simulink model "simulink_controller_3"  (R2020a)
settings: Solver=VariableStepAuto  StartTime=0.0  StopTime=10.0  RelTol=1e-3
libraries: simulink x2
settings Model: Creator=Jordan  LastModifiedBy=Jordan

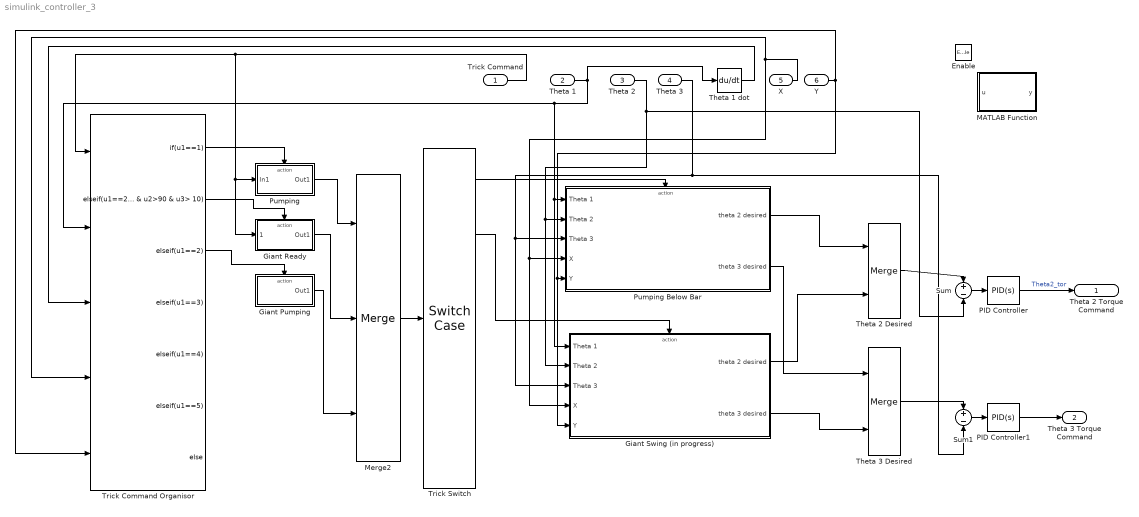
== system simulink_controller_3 ==
  "Trick Command " : Inport
  Theta 1 : Inport  Port=2
  Theta 2 : Inport  Port=3
  Theta 3 : Inport  Port=4
  X : Inport  Port=5
  Y : Inport  Port=6
  Enable : EnablePort
  Giant Pumping : Subsystem  TreatAsAtomicUnit=on
  Giant Ready : Subsystem  TreatAsAtomicUnit=on
  Giant Swing (in progress) : Subsystem  TreatAsAtomicUnit=on
  MATLAB Function : MATLAB Function  TreatAsAtomicUnit=on
  Merge2 : Merge  Inputs=3
  PID Controller : simulink/Continuous/PID Controller  Controller=PID  Form=Parallel  TimeDomain=Continuous-time  UseExternalTs=off  SampleTime=-1  IntegratorMethod=Forward Euler  FilterMethod=Forward Euler  ControllerParametersSource=internal  P=1  I=1  D=0  UseFilter=on  N=100  TunerSelectOption=Transfer Function Based (PID Tuner App)  InitialConditionSource=internal  InitialConditionForIntegrator=0  InitialConditionForFilter=0  DifferentiatorICPrevScaledInput=0  ExternalReset=none  TrackingMode=off  Kt=1  LimitOutput=off  UpperSaturationLimit=inf  LowerSaturationLimit=-inf  LinearizeAsGain=on  AntiWindupMode=none  Kb=1  POutMin=[]  POutMax=[]  IOutMin=[]  IOutMax=[]  DOutMin=[]  DOutMax=[]  NOutMin=[]  NOutMax=[]  SumOutMin=[]  SumOutMax=[]  SaturationOutMin=[]  SaturationOutMax=[]  PParamMin=[]  PParamMax=[]  IParamMin=[]  IParamMax=[]  DParamMin=[]  DParamMax=[]  NParamMin=[]  NParamMax=[]  KbParamMin=[]  KbParamMax=[]  KtParamMin=[]  KtParamMax=[]  KbOutMin=[]  KbOutMax=[]  KtOutMin=[]  KtOutMax=[]  IntegratorOutMin=[]  IntegratorOutMax=[]  FilterOutMin=[]  FilterOutMax=[]  SumI1OutMin=[]  SumI1OutMax=[]  SumI2OutMin=[]  SumI2OutMax=[]  SumI3OutMin=[]  SumI3OutMax=[]  SumI4OutMin=[]  SumI4OutMax=[]  SumDOutMin=[]  SumDOutMax=[]  DifferentiatorOutMin=[]  DifferentiatorOutMax=[]  FilterDiffOutCoefMin=[]  FilterDiffOutCoefMax=[]  ReciprocalOutMin=[]  ReciprocalOutMax=[]  SumDenOutMin=[]  SumDenOutMax=[]  SumNumOutMin=[]  SumNumOutMax=[]  DivideOutMin=[]  DivideOutMax=[]  UdiffTsProdOutMin=[]  UdiffTsProdOutMax=[]  NTsProdOutMin=[]  NTsProdOutMax=[]  UintegralTsProdOutMin=[]  UintegralTsProdOutMax=[]  UngainTsProdOutMin=[]  UngainTsProdOutMax=[]  IntegratorContinuousStateAttributes=''  IntegratorStateMustResolveToSignalObject=off  IntegratorRTWStateStorageClass=Auto  FilterContinuousStateAttributes=''  FilterStateMustResolveToSignalObject=off  FilterRTWStateStorageClass=Auto  ParallelPVariant=InternalParameters  IdealPVariant=Disabled  IVariant=InternalParameters  DVariant=InternalParameters  IntegratorVariant=Continuous  SatVariant=Disabled  AWVariant=Passthrough  PCopyVariant=Disabled  TRVariant=Disabled  FdbkBlocksVariant=Forward  IdealPFdbkVariant=Disabled  SatFdbkVariant=Disabled  DerivativeFilterVariant=ContFilter  NVariant=InternalParameters  NCopyVariant=Disabled  FilterICVariant=InternalICsFilter  IntegratorICVariant=InternalICs  ExternalResetVariant=Disabled  TRSumVariant=Passthrough  SumFdbkVariant=Disabled  SumVariant=Sum_PID  TsampFilterVariant=InternalTs  TsampNgainVariant=Passthrough  TsampIntegralVariant=Passthrough
  PID Controller1 : simulink/Continuous/PID Controller  Controller=PID  Form=Parallel  TimeDomain=Continuous-time  UseExternalTs=off  SampleTime=-1  IntegratorMethod=Forward Euler  FilterMethod=Forward Euler  ControllerParametersSource=internal  P=1  I=1  D=0  UseFilter=on  N=100  TunerSelectOption=Transfer Function Based (PID Tuner App)  InitialConditionSource=internal  InitialConditionForIntegrator=0  InitialConditionForFilter=0  DifferentiatorICPrevScaledInput=0  ExternalReset=none  TrackingMode=off  Kt=1  LimitOutput=off  UpperSaturationLimit=inf  LowerSaturationLimit=-inf  LinearizeAsGain=on  AntiWindupMode=none  Kb=1  POutMin=[]  POutMax=[]  IOutMin=[]  IOutMax=[]  DOutMin=[]  DOutMax=[]  NOutMin=[]  NOutMax=[]  SumOutMin=[]  SumOutMax=[]  SaturationOutMin=[]  SaturationOutMax=[]  PParamMin=[]  PParamMax=[]  IParamMin=[]  IParamMax=[]  DParamMin=[]  DParamMax=[]  NParamMin=[]  NParamMax=[]  KbParamMin=[]  KbParamMax=[]  KtParamMin=[]  KtParamMax=[]  KbOutMin=[]  KbOutMax=[]  KtOutMin=[]  KtOutMax=[]  IntegratorOutMin=[]  IntegratorOutMax=[]  FilterOutMin=[]  FilterOutMax=[]  SumI1OutMin=[]  SumI1OutMax=[]  SumI2OutMin=[]  SumI2OutMax=[]  SumI3OutMin=[]  SumI3OutMax=[]  SumI4OutMin=[]  SumI4OutMax=[]  SumDOutMin=[]  SumDOutMax=[]  DifferentiatorOutMin=[]  DifferentiatorOutMax=[]  FilterDiffOutCoefMin=[]  FilterDiffOutCoefMax=[]  ReciprocalOutMin=[]  ReciprocalOutMax=[]  SumDenOutMin=[]  SumDenOutMax=[]  SumNumOutMin=[]  SumNumOutMax=[]  DivideOutMin=[]  DivideOutMax=[]  UdiffTsProdOutMin=[]  UdiffTsProdOutMax=[]  NTsProdOutMin=[]  NTsProdOutMax=[]  UintegralTsProdOutMin=[]  UintegralTsProdOutMax=[]  UngainTsProdOutMin=[]  UngainTsProdOutMax=[]  IntegratorContinuousStateAttributes=''  IntegratorStateMustResolveToSignalObject=off  IntegratorRTWStateStorageClass=Auto  FilterContinuousStateAttributes=''  FilterStateMustResolveToSignalObject=off  FilterRTWStateStorageClass=Auto  ParallelPVariant=InternalParameters  IdealPVariant=Disabled  IVariant=InternalParameters  DVariant=InternalParameters  IntegratorVariant=Continuous  SatVariant=Disabled  AWVariant=Passthrough  PCopyVariant=Disabled  TRVariant=Disabled  FdbkBlocksVariant=Forward  IdealPFdbkVariant=Disabled  SatFdbkVariant=Disabled  DerivativeFilterVariant=ContFilter  NVariant=InternalParameters  NCopyVariant=Disabled  FilterICVariant=InternalICsFilter  IntegratorICVariant=InternalICs  ExternalResetVariant=Disabled  TRSumVariant=Passthrough  SumFdbkVariant=Disabled  SumVariant=Sum_PID  TsampFilterVariant=InternalTs  TsampNgainVariant=Passthrough  TsampIntegralVariant=Passthrough
  Pumping : Subsystem  TreatAsAtomicUnit=on
  Pumping Below Bar : Subsystem  TreatAsAtomicUnit=on
  Sum : Sum  Inputs=+-
  Sum1 : Sum  Inputs=+-
  Theta 1 dot : Derivative
  Theta 2 Desired : Merge
  Theta 3 Desired : Merge
  Trick Command Organisor : If  NumInputs=5  IfExpression=u1==1  ElseIfExpressions=u1==2 & u2>90 & u3> 10, u1==2, u1==3, u1==4, u1==5
  Trick Switch : SwitchCase  CaseConditions={1,2,3,4,5}
  Theta 2 Torque Command : Outport
  Theta 3 Torque Command : Outport  Port=2
  wires:
  Theta 2 Desired/1 -> Sum/1
  Theta 3 Desired/1 -> Sum1/1
  Giant Swing (in progress)/1(theta 2 desired) -> Theta 2 Desired/2
  Trick Switch/2 -> Giant Swing (in progress)/Action
  Pumping Below Bar/2(theta 3 desired) -> Theta 3 Desired/1
  Giant Swing (in progress)/2(theta 3 desired) -> Theta 3 Desired/2
  Pumping Below Bar/1(theta 2 desired) -> Theta 2 Desired/1
  Trick Switch/1 -> Pumping Below Bar/Action
  "Trick Command "/1 -> Giant Ready/1(" "), Pumping/1(In1), Trick Command Organisor/1
  Theta 2/1 -> Sum/2, Giant Swing (in progress)/2(Theta 2), Pumping Below Bar/2(Theta 2)
  Theta 3/1 -> Sum1/2, Pumping Below Bar/3(Theta 3), Giant Swing (in progress)/3(Theta 3)
  X/1 -> Trick Command Organisor/4, Giant Swing (in progress)/4(X), Pumping Below Bar/4(X)
  Y/1 -> Trick Command Organisor/5, Giant Swing (in progress)/5(Y), Pumping Below Bar/5(Y)
  Theta 1/1 -> Giant Swing (in progress)/1(Theta 1), Pumping Below Bar/1(Theta 1), Trick Command Organisor/2, Theta 1 dot/1
  Theta 1 dot/1 -> Trick Command Organisor/3
  Merge2/1 -> Trick Switch/1
  Trick Command Organisor/1 -> Pumping/Action
  Pumping/1(Out1) -> Merge2/1
  Trick Command Organisor/2 -> Giant Ready/Action
  Giant Ready/1(Out1) -> Merge2/2
  Trick Command Organisor/3 -> Giant Pumping/Action
  Giant Pumping/1(Out1) -> Merge2/3
  PID Controller/1 -> Theta 2 Torque Command/1  "Theta2_tor"
  PID Controller1/1 -> Theta 3 Torque Command/1
  Sum/1 -> PID Controller/1
  Sum1/1 -> PID Controller1/1
  ? -> ?

== system simulink_controller_3/Giant Pumping ==
  Action Port : ActionPort  ActionPortLabel=elseif( u1==2)
  Constant : Constant
  Out1 : Outport
  wires:
  Constant/1 -> Out1/1

== system simulink_controller_3/Giant Ready ==
  " " : Inport
  Action Port : ActionPort  ActionPortLabel=elseif(u1==2 & u2>90 & u3> 10)
  Out1 : Outport
  wires:
  " "/1 -> Out1/1

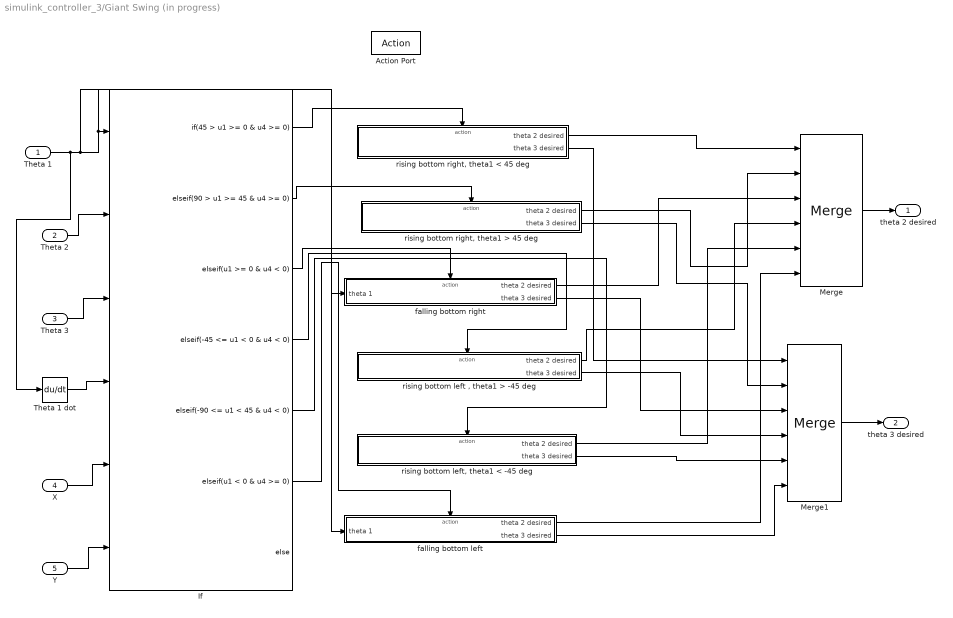
== system simulink_controller_3/Giant Swing (in progress) ==
  Theta 1 : Inport
  Theta 2 : Inport  Port=2
  Theta 3 : Inport  Port=3
  X : Inport  Port=4
  Y : Inport  Port=5
  Action Port : ActionPort  ActionPortLabel=case [ 2 ]:
  If : If  NumInputs=6  IfExpression=45 > u1 >= 0 & u4 >= 0  ElseIfExpressions="90 > u1 >= 45 & u4 >= 0, u1 >= 0 & u4 < 0, -45 <= u1 < 0 & u4 < 0, -90 <= u1 < 45 & u4 < 0,  u1 < 0 & u4 >= 0"
  Merge : Merge  Inputs=6
  Merge1 : Merge  Inputs=6
  Theta 1 dot : Derivative
  falling bottom left : Subsystem  TreatAsAtomicUnit=on
  falling bottom right : Subsystem  TreatAsAtomicUnit=on
  "rising bottom left , theta1 > -45 deg" : Subsystem  TreatAsAtomicUnit=on
  "rising bottom left, theta1 < -45 deg" : Subsystem  TreatAsAtomicUnit=on
  "rising bottom right, theta1 < 45 deg" : Subsystem  TreatAsAtomicUnit=on
  "rising bottom right, theta1 > 45 deg" : Subsystem  TreatAsAtomicUnit=on
  theta 2 desired : Outport
  theta 3 desired : Outport  Port=2
  wires:
  "rising bottom left, theta1 < -45 deg"/1(theta 2 desired) -> Merge/5
  If/4 -> "rising bottom left , theta1 > -45 deg"/Action
  "rising bottom left, theta1 < -45 deg"/2(theta 3 desired) -> Merge1/5
  falling bottom left/2(theta 3 desired) -> Merge1/6
  X/1 -> If/5
  If/5 -> "rising bottom left, theta1 < -45 deg"/Action
  "rising bottom right, theta1 > 45 deg"/2(theta 3 desired) -> Merge1/2
  falling bottom left/1(theta 2 desired) -> Merge/6
  If/2 -> "rising bottom right, theta1 > 45 deg"/Action
  "rising bottom left , theta1 > -45 deg"/2(theta 3 desired) -> Merge1/4
  "rising bottom right, theta1 < 45 deg"/1(theta 2 desired) -> Merge/1
  If/6 -> falling bottom left/Action
  "rising bottom right, theta1 < 45 deg"/2(theta 3 desired) -> Merge1/1
  "rising bottom right, theta1 > 45 deg"/1(theta 2 desired) -> Merge/2
  Merge/1 -> theta 2 desired/1
  Merge1/1 -> theta 3 desired/1
  If/1 -> "rising bottom right, theta1 < 45 deg"/Action
  Theta 1 dot/1 -> If/4
  Theta 1/1 -> Theta 1 dot/1, falling bottom right/1(theta 1), falling bottom left/1(theta 1), If/1
  falling bottom right/1(theta 2 desired) -> Merge/3
  "rising bottom left , theta1 > -45 deg"/1(theta 2 desired) -> Merge/4
  Y/1 -> If/6
  Theta 3/1 -> If/3
  falling bottom right/2(theta 3 desired) -> Merge1/3
  If/3 -> falling bottom right/Action
  Theta 2/1 -> If/2

== system simulink_controller_3/Pumping ==
  In1 : Inport
  Action Port : ActionPort  ActionPortLabel=if(u1==1)
  Out1 : Outport
  wires:
  In1/1 -> Out1/1

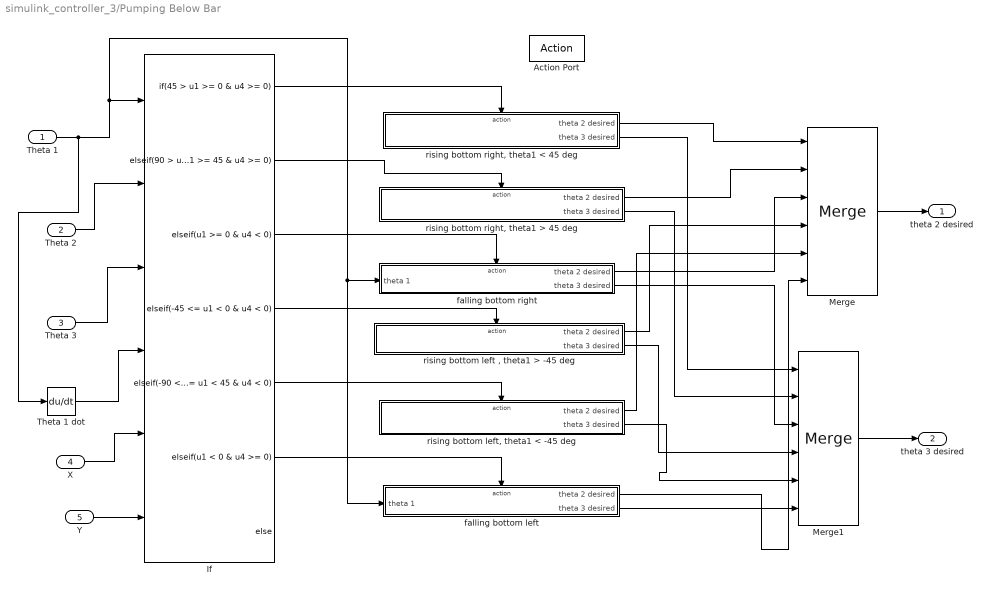
== system simulink_controller_3/Pumping Below Bar ==
  Theta 1 : Inport
  Theta 2 : Inport  Port=2
  Theta 3 : Inport  Port=3
  X : Inport  Port=4
  Y : Inport  Port=5
  Action Port : ActionPort  ActionPortLabel=case [ 1 ]:
  If : If  NumInputs=6  IfExpression=45 > u1 >= 0 & u4 >= 0  ElseIfExpressions="90 > u1 >= 45 & u4 >= 0, u1 >= 0 & u4 < 0, -45 <= u1 < 0 & u4 < 0, -90 <= u1 < 45 & u4 < 0,  u1 < 0 & u4 >= 0"
  Merge : Merge  Inputs=6
  Merge1 : Merge  Inputs=6
  Theta 1 dot : Derivative
  falling bottom left : Subsystem  TreatAsAtomicUnit=on
  falling bottom right : Subsystem  TreatAsAtomicUnit=on
  "rising bottom left , theta1 > -45 deg" : Subsystem  TreatAsAtomicUnit=on
  "rising bottom left, theta1 < -45 deg" : Subsystem  TreatAsAtomicUnit=on
  "rising bottom right, theta1 < 45 deg" : Subsystem  TreatAsAtomicUnit=on
  "rising bottom right, theta1 > 45 deg" : Subsystem  TreatAsAtomicUnit=on
  theta 2 desired : Outport
  theta 3 desired : Outport  Port=2
  wires:
  "rising bottom left, theta1 < -45 deg"/1(theta 2 desired) -> Merge/5
  If/4 -> "rising bottom left , theta1 > -45 deg"/Action
  "rising bottom left, theta1 < -45 deg"/2(theta 3 desired) -> Merge1/5
  falling bottom left/2(theta 3 desired) -> Merge1/6
  X/1 -> If/5
  If/5 -> "rising bottom left, theta1 < -45 deg"/Action
  "rising bottom right, theta1 > 45 deg"/2(theta 3 desired) -> Merge1/2
  falling bottom left/1(theta 2 desired) -> Merge/6
  If/2 -> "rising bottom right, theta1 > 45 deg"/Action
  "rising bottom left , theta1 > -45 deg"/2(theta 3 desired) -> Merge1/4
  "rising bottom right, theta1 < 45 deg"/1(theta 2 desired) -> Merge/1
  If/6 -> falling bottom left/Action
  "rising bottom right, theta1 < 45 deg"/2(theta 3 desired) -> Merge1/1
  "rising bottom right, theta1 > 45 deg"/1(theta 2 desired) -> Merge/2
  Merge/1 -> theta 2 desired/1
  Merge1/1 -> theta 3 desired/1
  If/1 -> "rising bottom right, theta1 < 45 deg"/Action
  Theta 1 dot/1 -> If/4
  Theta 1/1 -> Theta 1 dot/1, falling bottom right/1(theta 1), falling bottom left/1(theta 1), If/1
  falling bottom right/1(theta 2 desired) -> Merge/3
  "rising bottom left , theta1 > -45 deg"/1(theta 2 desired) -> Merge/4
  Y/1 -> If/6
  Theta 3/1 -> If/3
  falling bottom right/2(theta 3 desired) -> Merge1/3
  If/3 -> falling bottom right/Action
  Theta 2/1 -> If/2

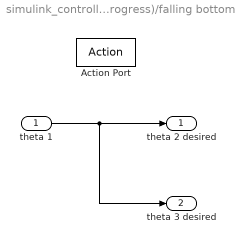
== system simulink_controller_3/Giant Swing (in progress)/falling bottom left ==
  theta 1 : Inport
  Action Port : ActionPort  ActionPortLabel="elseif(  u1 < 0 & u4 >= 0)"
  theta 2 desired : Outport
  theta 3 desired : Outport  Port=2
  wires:
  theta 1/1 -> theta 3 desired/1, theta 2 desired/1

== system simulink_controller_3/Giant Swing (in progress)/falling bottom right ==
  theta 1 : Inport
  Action Port : ActionPort  ActionPortLabel=elseif( u1 >= 0 & u4 < 0)
  theta 2 desired : Outport
  theta 3 desired : Outport  Port=2
  wires:
  theta 1/1 -> theta 3 desired/1, theta 2 desired/1

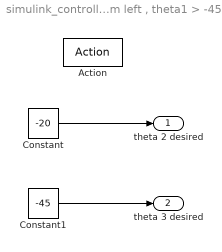
== system simulink_controller_3/Giant Swing (in progress)/rising bottom left , theta1 > -45 deg ==
  Action : ActionPort  ActionPortLabel=elseif( -45 <= u1 < 0 & u4 < 0)
  Constant : Constant  Value=-20
  Constant1 : Constant  Value=-45
  theta 2 desired : Outport
  theta 3 desired : Outport  Port=2
  wires:
  Constant/1 -> theta 2 desired/1
  Constant1/1 -> theta 3 desired/1

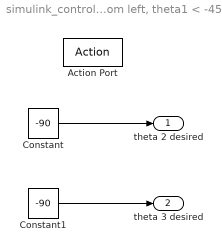
== system simulink_controller_3/Giant Swing (in progress)/rising bottom left, theta1 < -45 deg ==
  Action Port : ActionPort  ActionPortLabel=elseif( -90 <= u1 < 45 & u4 < 0)
  Constant : Constant  Value=-90
  Constant1 : Constant  Value=-90
  theta 2 desired : Outport
  theta 3 desired : Outport  Port=2
  wires:
  Constant/1 -> theta 2 desired/1
  Constant1/1 -> theta 3 desired/1

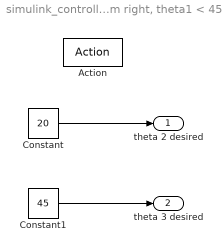
== system simulink_controller_3/Giant Swing (in progress)/rising bottom right, theta1 < 45 deg ==
  Action : ActionPort  ActionPortLabel=if(45 > u1 >= 0 & u4 >= 0)
  Constant : Constant  Value=20
  Constant1 : Constant  Value=45
  theta 2 desired : Outport
  theta 3 desired : Outport  Port=2
  wires:
  Constant/1 -> theta 2 desired/1
  Constant1/1 -> theta 3 desired/1

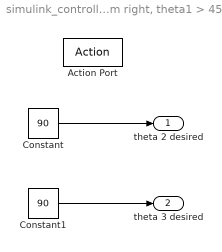
== system simulink_controller_3/Giant Swing (in progress)/rising bottom right, theta1 > 45 deg ==
  Action Port : ActionPort  ActionPortLabel=elseif(90 > u1 >= 45 & u4 >= 0)
  Constant : Constant  Value=90
  Constant1 : Constant  Value=90
  theta 2 desired : Outport
  theta 3 desired : Outport  Port=2
  wires:
  Constant/1 -> theta 2 desired/1
  Constant1/1 -> theta 3 desired/1

== system simulink_controller_3/Pumping Below Bar/falling bottom left ==
  theta 1 : Inport
  Action Port : ActionPort  ActionPortLabel="elseif(  u1 < 0 & u4 >= 0)"
  theta 2 desired : Outport
  theta 3 desired : Outport  Port=2
  wires:
  theta 1/1 -> theta 3 desired/1, theta 2 desired/1

== system simulink_controller_3/Pumping Below Bar/falling bottom right ==
  theta 1 : Inport
  Action Port : ActionPort  ActionPortLabel=elseif( u1 >= 0 & u4 < 0)
  theta 2 desired : Outport
  theta 3 desired : Outport  Port=2
  wires:
  theta 1/1 -> theta 3 desired/1, theta 2 desired/1

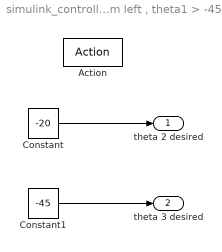
== system simulink_controller_3/Pumping Below Bar/rising bottom left , theta1 > -45 deg ==
  Action : ActionPort  ActionPortLabel=elseif( -45 <= u1 < 0 & u4 < 0)
  Constant : Constant  Value=-20
  Constant1 : Constant  Value=-45
  theta 2 desired : Outport
  theta 3 desired : Outport  Port=2
  wires:
  Constant/1 -> theta 2 desired/1
  Constant1/1 -> theta 3 desired/1

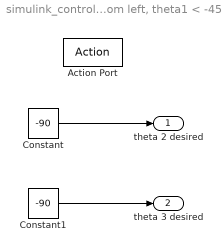
== system simulink_controller_3/Pumping Below Bar/rising bottom left, theta1 < -45 deg ==
  Action Port : ActionPort  ActionPortLabel=elseif( -90 <= u1 < 45 & u4 < 0)
  Constant : Constant  Value=-90
  Constant1 : Constant  Value=-90
  theta 2 desired : Outport
  theta 3 desired : Outport  Port=2
  wires:
  Constant/1 -> theta 2 desired/1
  Constant1/1 -> theta 3 desired/1

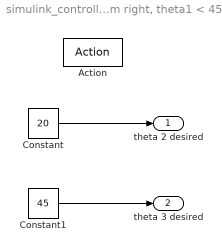
== system simulink_controller_3/Pumping Below Bar/rising bottom right, theta1 < 45 deg ==
  Action : ActionPort  ActionPortLabel=if(45 > u1 >= 0 & u4 >= 0)
  Constant : Constant  Value=20
  Constant1 : Constant  Value=45
  theta 2 desired : Outport
  theta 3 desired : Outport  Port=2
  wires:
  Constant/1 -> theta 2 desired/1
  Constant1/1 -> theta 3 desired/1

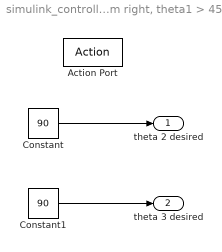
== system simulink_controller_3/Pumping Below Bar/rising bottom right, theta1 > 45 deg ==
  Action Port : ActionPort  ActionPortLabel=elseif(90 > u1 >= 45 & u4 >= 0)
  Constant : Constant  Value=90
  Constant1 : Constant  Value=90
  theta 2 desired : Outport
  theta 3 desired : Outport  Port=2
  wires:
  Constant/1 -> theta 2 desired/1
  Constant1/1 -> theta 3 desired/1

== matlab function simulink_controller_3/MATLAB Function ==
  data: u input; y output
function y = fcn(u)
main_uneven_on_bar();
y = u;
